simulink library "libResultDataStorer"  (R2020b)
settings: Solver=VariableStepAuto  StartTime=0.0  StopTime=10.0  RelTol=1e-3
settings Model: Creator=caatay  LastModifiedBy=caatay

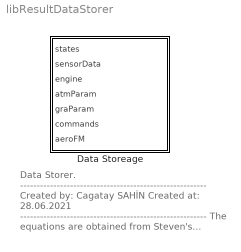
== system libResultDataStorer ==
  note: Data Storer.
      | --------------------------------------------------------
      | Created by: Cagatay SAHİN
      | Created at: 28.06.2021
      | --------------------------------------------------------
      | The equations are obtained from
      | Steven's textbook.
      | The reference book can be found in
      | "references folder".
      | --------------------------------------------------------
      | for question:
      | cagataysahin44@gmail.com
  Data Storeage : Subsystem  mask(Flight Control System - Data Storer){}
      mask help: Simulation Result data storere to obtain wholoe simulation data in MATLAB.
      mask Help:
      | This block integrate state derivative to state variables.
      | -------------------------------------------------------------------------------------------------------------------------------------------------
      | Inputs of this block set are:
      | 	states: Information of state variables.
      | 	sensorData: Information of sensor data.
      | 	engine: Information of engine.
      | 	atm: Information of atmosphere parameters.
      | 	gravity: Information of gravity Parameters.
      | 	commands: Information of pilot commands and flight surfaces
      | 	aeroFM: Information of aerodynamic forces and moments
      | -------------------------------------------------------------------------------------------------------------------------------------------------
      | For question: "cagataysahin44@gmail.com"
      mask Display:
      | port_label('input',1,'Inf_{states}','texmode','on');
      | port_label('input',2,'Inf_{sensor}','texmode','on');
      | port_label('input',3,'Inf_{engine}','texmode','on');
      | port_label('input',4,'Inf_{atm}','texmode','on');
      | port_label('input',5,'Inf_{gravity}','texmode','on');
      | port_label('input',6,'Inf_{commands}','texmode','on');
      | port_label('input',7,'Inf_{aeroFM}','texmode','on');

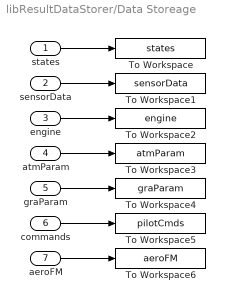
== system libResultDataStorer/Data Storeage ==
  states : Inport
  sensorData : Inport  Port=2
  engine : Inport  Port=3
  atmParam : Inport  Port=4
  graParam : Inport  Port=5
  commands : Inport  Port=6
  aeroFM : Inport  Port=7
  To Workspace : ToWorkspace  VariableName=states  SampleTime=-1
      settings: Save2DSignal=2-D array (concatenate along first dimension)
  To Workspace1 : ToWorkspace  VariableName=sensorData  SampleTime=-1
      settings: Save2DSignal=2-D array (concatenate along first dimension)
  To Workspace2 : ToWorkspace  VariableName=engine  SampleTime=-1
      settings: Save2DSignal=2-D array (concatenate along first dimension)
  To Workspace3 : ToWorkspace  VariableName=atmParam  SampleTime=-1
      settings: Save2DSignal=2-D array (concatenate along first dimension)
  To Workspace4 : ToWorkspace  VariableName=graParam  SampleTime=-1
      settings: Save2DSignal=2-D array (concatenate along first dimension)
  To Workspace5 : ToWorkspace  VariableName=pilotCmds  SampleTime=-1
      settings: Save2DSignal=2-D array (concatenate along first dimension)
  To Workspace6 : ToWorkspace  VariableName=aeroFM  SampleTime=-1
      settings: Save2DSignal=2-D array (concatenate along first dimension)
  wires:
  states/1 -> To Workspace/1
  sensorData/1 -> To Workspace1/1
  engine/1 -> To Workspace2/1
  atmParam/1 -> To Workspace3/1
  graParam/1 -> To Workspace4/1
  commands/1 -> To Workspace5/1
  aeroFM/1 -> To Workspace6/1
